simulink model "RASCAL72_cl"  (R2017b)
settings: Solver=FixedStepDiscrete  StartTime=0.0  StopTime=100  RelTol=1e-3  EnableMultiTasking=on
values from neighbouring files (symbols this model uses):
  CD0 = 0.0164    [Final_Project_START.m]
  CDa_200 = [0.53 0.53 0.53 0.53 0.53 0.53 0.53 0.53 0.53 0.53 0.53 0.53 ... (25 elements, 5x5)]    [C1o_200.mat]    (also in CDa_200.mat; CLadot_200.mat; CLde.mat; CLo_200.mat)
  CDde_200 = [0 0 0 0 0 0 0 0 0 0 0 0 ... (25 elements, 5x5)]    [C1o_200.mat]    (also in CDde_200.mat; CLadot_200.mat; CLde.mat; CLo_200.mat)
  CDq_200 = [0 0 0 0 0 0 0 0 0 0 0 0 ... (25 elements, 5x5)]    [C1o_200.mat]    (also in CDq_200.mat; CLadot_200.mat; CLde.mat; CLo_200.mat)
  CL0 = 0.21    [Final_Project_START.m]
  Cl0 = 0    [Final_Project_START.m]
  CLa_200 = [5.326215664 5.440234265 5.741037107 5.849899088 5.539928921 5.331372284 5.445390885 5.746766685 5.849899088 5.539355963 5.335955946 5.449401589 ... (25 elements, 5x5)]    [C1o_200.mat]    (also in CLa_200.mat; CLadot_200.mat; CLde.mat; CLo_200.mat)
  ClB_200 = [-0.052500123 -0.052614714 -0.052614714 -0.05294703 -0.053136106 -0.052523041 -0.052649092 -0.052666281 -0.053015785 -0.05322205 -0.052545959 -0.0525345 ... (25 elements, 5x5)]    [C1B_200.mat]    (also in C1o_200.mat; CLadot_200.mat; Cma_200.mat; Cmadot_200.mat)
  Clda_200 = [0.03678389 0.037299552 0.037299552 0.036726595 0.035580679 0.03678389 0.037299552 0.037299552 0.036726595 0.035580679 0.03678389 0.037299552 ... (25 elements, 5x5)]    [C1da_200.mat]    (also in C1o_200.mat = [0.000642 0.000651 0.000651 0.000641 0.000621 0.000642 0.000; CLadot_200.mat = [0.000642 0.000651 0.000651 0.000641 0.000621 0.000642 0.000; Cma_200.mat = [0.000642 0.000651 0.000651 0.000641 0.000621 0.000642 0.000; Cmadot_200.mat = [0.000642 0.000651 0.000651 0.000641 0.000621 0.000642 0.000)
  CLde_200 = [0.001609 0.00164 0.001639 0.001604 0.001542 0.001609 0.00164 0.001639 0.001604 0.001542 0.001609 0.00164 ... (25 elements, 5x5)]    [C1o_200.mat]    (also in CLadot_200.mat; CLde.mat; CLde_200.mat = [0.092188909 0.093965078 0.093907783 0.09190243 0.088350092 ; CLo_200.mat)
  Cldr_200 = [-5.72958e-05 0 5.72958e-05 0.000114592 0.000171887 -5.72958e-05 0 5.72958e-05 0.000114592 0.000171887 -5.72958e-05 0 ... (25 elements, 5x5)]    [C1dr_200.mat]    (also in C1o_200.mat = [-1e-06 0 1e-06 2e-06 3e-06 -1e-06 0 1e-06 2e-06 3e-06 -1e-0; CLadot_200.mat = [-1e-06 0 1e-06 2e-06 3e-06 -1e-06 0 1e-06 2e-06 3e-06 -1e-0; Cma_200.mat = [-1e-06 0 1e-06 2e-06 3e-06 -1e-06 0 1e-06 2e-06 3e-06 -1e-0; Cmadot_200.mat = [-1e-06 0 1e-06 2e-06 3e-06 -1e-06 0 1e-06 2e-06 3e-06 -1e-0)
  Clp_200 = [-0.448740545 -0.460829955 -0.490337281 -0.496124155 -0.462205053 -0.448740545 -0.460772659 -0.490279985 -0.496009563 -0.461861279 -0.448797841 -0.460829955 ... (25 elements, 5x5)]    [C1o_200.mat]    (also in C1p_200.mat; CLadot_200.mat; Cma_200.mat; Cmadot_200.mat)
  CLq_200 = [9.310564171 9.310564171 9.310564171 9.310564171 9.310564171 9.344941639 9.344941639 9.344941639 9.344941639 9.344941639 9.373589528 9.373589528 ... (25 elements, 5x5)]    [C1o_200.mat]    (also in CLadot_200.mat; CLde.mat; CLo_200.mat; CLq_200.mat)
  Clr_200 = [-0.074885584 0.016254813 0.110122488 0.213369483 0.308595068 -0.07494288 0.016260542 0.11023708 0.21354137 0.308824252 -0.075000175 0.016272001 ... (25 elements, 5x5)]    [C1o_200.mat]    (also in C1r_200.mat; CLadot_200.mat; CLde.mat; CLo_200.mat)
  Cm0 = 0    [Final_Project_START.m]
  Cma_200 = [-1.61689 -1.94061 -2.12224 -2.54508 -2.95302 -1.61918 -1.94978 -2.1314 -2.55367 -2.96506 -1.62319 -1.9578 ... (25 elements, 5x5)]    [C1o_200.mat]    (also in CLadot_200.mat; CLde.mat; CLo_200.mat; CLq_200.mat)
  Cmde_200 = [-0.002239 -0.002272 -0.00227 -0.00223 -0.002161 -0.002239 -0.002272 -0.00227 -0.00223 -0.002161 -0.002239 -0.002272 ... (25 elements, 5x5)]    [C1o_200.mat]    (also in CLadot_200.mat; CLde.mat; CLo_200.mat; CLq_200.mat)
  Cmq_200 = [-17.06841272 -17.06841272 -17.06841272 -17.06841272 -17.06841272 -17.17154512 -17.17154512 -17.17154512 -17.17154512 -17.17154512 -17.25175921 -17.25175921 ... (25 elements, 5x5)]    [C1o_200.mat]    (also in CLadot_200.mat; CLde.mat; CLo_200.mat; CLq_200.mat)
  Cn0 = 0    [Final_Project_START.m]
  CnB_200 = [0.029759428 0.029759428 0.029759428 0.029759428 0.029759428 0.028264008 0.028264008 0.028264008 0.028264008 0.028264008 0.027209766 0.027209766 ... (25 elements, 5x5)]    [C1o_200.mat]    (also in CLadot_200.mat; CLde.mat; CLo_200.mat; CLq_200.mat)
  Cnda_200 = [-4.5e-05 -2.9e-05 -1.1e-05 6e-06 2.2e-05 -4.5e-05 -2.9e-05 -1.1e-05 6e-06 2.2e-05 -4.5e-05 -2.9e-05 ... (25 elements, 5x5)]    [C1o_200.mat]    (also in CLadot_200.mat; CLde.mat; CLo_200.mat; CLq_200.mat)
  Cndr_200 = [0.000151 0.000159 0.000163 0.000164 0.00016 0.000151 0.000159 0.000163 0.000164 0.00016 0.000151 0.000159 ... (25 elements, 5x5)]    [C1o_200.mat]    (also in CLadot_200.mat; CLde.mat; CLo_200.mat; CLq_200.mat)
  Cnp_200 = [0.038193 0.000534 -0.03759 -0.07993 -0.12032 0.039712 0.000373 -0.03967 -0.08394 -0.12594 0.040583 0.00028 ... (25 elements, 5x5)]    [C1o_200.mat]    (also in CLadot_200.mat; CLde.mat; CLo_200.mat; CLq_200.mat)
  Cnr_200 = [-0.040473739 -0.043229666 -0.042771299 -0.038405361 -0.030859507 -0.040015372 -0.042908809 -0.042244178 -0.037247986 -0.028751022 -0.039728894 -0.042702544 ... (25 elements, 5x5)]    [C1o_200.mat]    (also in CLadot_200.mat; CLde.mat; CLo_200.mat; CLq_200.mat)
  CY0 = 0    [Final_Project_START.m]
  CYB_200 = [-0.504374747 -0.504374747 -0.504374747 -0.504374747 -0.504374747 -0.504374747 -0.504374747 -0.504374747 -0.504374747 -0.504374747 -0.504432043 -0.50432043 ... (25 elements, 5x5)]    [C1o_200.mat]    (also in CLadot_200.mat; CLde.mat; CLo_200.mat; CLq_200.mat)
  CYda_200 = [4e-06 2.7e-05 5e-05 7.1e-05 9.1e-05 4e-06 2.7e-05 5e-05 7.1e-05 9.1e-05 4e-06 2.7e-05 ... (25 elements, 5x5)]    [C1o_200.mat]    (also in CLadot_200.mat; CLde.mat; CLo_200.mat; CLq_200.mat)
  CYdr_200 = [-0.000731 -0.000766 -0.000782 -0.00078 -0.000759 -0.000731 -0.000766 -0.000782 -0.00078 -0.000759 -0.000731 -0.000766 ... (25 elements, 5x5)]    [C1o_200.mat]    (also in CLadot_200.mat; CLde.mat; CLo_200.mat; CLq_200.mat)
  CYp_200 = [-0.030521462 -0.058498991 -0.087204176 -0.119576292 -0.14919821 -0.029782346 -0.058613582 -0.088178205 -0.121581644 -0.152005703 -0.029358357 -0.058670878 ... (25 elements, 5x5)]    [C1o_200.mat]    (also in CLadot_200.mat; CLde.mat; CLo_200.mat; CLq_200.mat)
  CYr_200 = [0.026877 0.03248 0.035656 0.0363 0.03441 0.026877 0.03248 0.035656 0.0363 0.03441 0.026877 0.03248 ... (25 elements, 5x5)]    [C1o_200.mat]    (also in CLadot_200.mat; CLde.mat; CLo_200.mat; CLq_200.mat)
undefined symbols (not defined in the file or in its folder): airlib, B747, DiscIntNeverNeededParam, DT
(part 1 of 2)
settings Model: Creator=SHETTYA1  LastModifiedBy=antar
settings DataIOCC: SaveFormat=Array  SignalLoggingSaveFormat=ModelDataLogs  SaveOutput=off  SaveTime=off
settings OptimizationCC: BlockReduction=off  BooleanDataType=off
settings DebuggingCC: SaveWithParameterizedLinksMsg=none  UnderspecifiedInitializationDetection=Classic  MergeDetectMultiDrivingBlocksExec=none  SignalResolutionControl=TryResolveAllWithWarning  MultiTaskDSMMsg=warning  MultiTaskCondExecSysMsg=none
settings HardwareCC: TargetUnknown=on
settings ModelReferenceCC: PropagateSignalLabelsOutOfModel=off
settings CodeAppCC: StateflowObjectComments=on
settings GRTTargetCC: TargetLangStandard=C89/C90 (ANSI)  CombineOutputUpdateFcns=off  GRTInterface=on

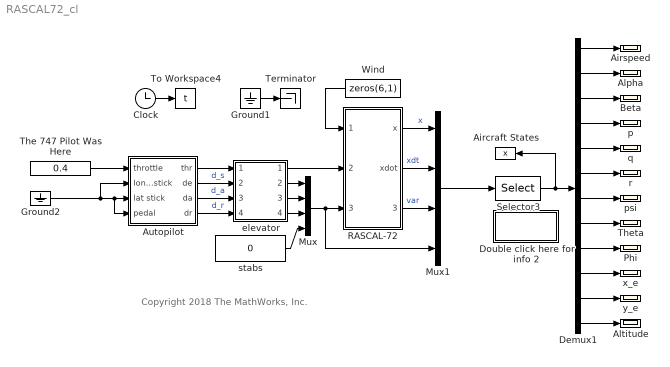
== system RASCAL72_cl ==
  note: Copyright 2018 The MathWorks, Inc.
  Aircraft States : ToWorkspace  VariableName=x  SampleTime=0.05
  Airspeed : Scope
  Alpha : Scope
  Altitude : Scope
  Autopilot : Subsystem
  Beta : Scope
  Clock : Clock
  Demux1 : Demux  Outputs=12
  Double click here for info 2 : Subsystem
      mask Display: disp('Output\nSignals')
  Ground1 : Ground
  Ground2 : Ground
  Mux : Mux
  Mux1 : Mux  Inputs=[12 12 12 4]
  Phi : Scope
  RASCAL-72 : Subsystem  AncestorBlock=airlib/DT-B747  mask(Discrete Time General Nonlinear Aircraft Model){GM1=[0.244   1.84   0.327418   1.7398  1.3865   1.7122   0   0  0   2.9  0.05], CD_wind=[0.076   0.53  0  0  0], CL_wind=[0.2  5.849899088  9.310  0.001604  0], Cm_body=[0.3567  -2.54508  -17.0684   -7.288023154    0], CY_body=[0   -0.504374747  -0.119633588   0.0363     0.000071  -0.00078  ], Cl_body=[0  -0.05294703   -0.496124155    0.213369  0.000641  0.000002], Cn_body=[0 0.029747969 -0.07993 -0.038399631 0.000006 0.000164], x0=[10 0.0264  0   0 0 0   0  0.08  0   0 0 100]}
      mask prompts: GM1 "Geometry, Mass, T : [cbar   b    S    Ix   Iy   Iz   Jxy  Jxz  Jyz  m  T]"; CD_wind "Aerodynamic D-Force Derivatives : [CD0 CDa CDq CDde CDih]"; CL_wind "Aerodynamic L-Force Derivatives : [CL0 CLa CLq CLde CLih]"; Cm_body "Aerodynamic Y-Moment Derivatives : [Cm0 Cma Cmq Cmde Cmih]"; CY_body "Aerodynamic Y-Force Derivatives : [CY0 CYb CYp CYr CYda CYdr]"; Cl_body "Aerodynamic X-moment Derivatives : [Cl0 Clb Clp Clr Clda Cldr]"; Cn_body "Aerodynamic Z-moment Derivatives : [Cn0 Cnb Cnp Cnr Cnda Cndr]"; x0 "Initial Condition x0 [v alpha beta p q r psi theta phi xe ye H]"
      mask help:
      | The first input contains the wind velocity and acceleration.The second input contains external forces and moments in body axis. The third input contains the deflections of elevators, ailerons, rudder, and flaps. For explanations about outputs and parameters open the help and/or look under the mask.
      | The International measurement system (MKS) is adopted.
      mask init:
      | AM=zeros(6,19);
      | AM(1,[1 2 9 11 12])=reshape(CD_wind,1,5);
      | AM(3,[1 2 9 11 12])=reshape(CL_wind,1,5);
      | AM(5,[1 2 9 11 12])=reshape(Cm_body,1,5);
      | AM(2,[1 5 8 10 13 14])=reshape(CY_body,1,6);
      | AM(4,[1 5 8 10 13 14])=reshape(Cl_body,1,6);
      | AM(6,[1 5 8 10 13 14])=reshape(Cn_body,1,6);
      | 
      | Ix=GM1(4);Iy=GM1(5);Iz=GM1(6);
      | Jxy=GM1(7);Jxz=GM1(8);Jyz=GM1(9);
      | 
      | detI = Ix*Iy*Iz - 2*Jxy*Jxz*Jyz - Ix*Jyz^2 - Iy*Jxz^2 - Iz*Jxy^2;
      | I1   = Iy*Iz - Jyz^2;I2   = Jxy*Iz + Jyz*Jxz;
      | I3   = Jxy*Jyz + Iy*Jxz;I4   = Ix*Iz - Jxz^2;
      | I5   = Ix*Jyz + Jxy*Jxz;I6   = Ix*Iy - Jxy^2;
      | 
      | Pl  = I1/detI; Pm = I2/detI; Pn = I3/detI;
      | Ppp = -(Jxz*I2 - Jxy*I3)/detI;Ppq = (Jxz*I1 - Jyz*I2 - (Iy-Ix)*I3)/detI;
      | Ppr = -(Jxy*I1 + (Ix-Iz)*I2 - Jyz*I3)/detI;Pqq = (Jyz*I1 - Jxy*I3)/detI;
      | Pqr = -((Iz-Iy)*I1 - Jxy*I2 + Jxz*I3)/detI;Prr = -(Jyz*I1 - Jxz*I2)/detI;
      | 
      | Ql  = I2/detI; Qm = I4/detI; Qn = I5/detI;
      | Qpp = -(Jxz*I4 - Jxy*I5)/detI;Qpq = (Jxz*I2 - Jyz*I4 - (Iy-Ix)*I5)/detI;
      | Qpr = -(Jxy*I2 + (Ix-Iz)*I4 - Jyz*I5)/detI;Qqq = (Jyz*I2 - Jxy*I5)/detI;
      | Qqr = -((Iz-Iy)*I2 - Jxy*I4 + Jxz*I5)/detI;Qrr = -(Jyz*I2 - Jxz*I4)/detI;
      | 
      | Rl  = I3/detI; Rm = I5/detI; Rn = I6/detI;
      | Rpp = -(Jxz*I5 - Jxy*I6)/detI;
      | Rpq = (Jxz*I3 - Jyz*I5 - (Iy-Ix)*I6)/detI;
      | Rpr = -(Jxy*I3 + (Ix-Iz)*I5 - Jyz*I6)/detI;
      | Rqq = (Jyz*I3 - Jxy*I6)/detI;
      | Rqr = -((Iz-Iy)*I3 - Jxy*I5 + Jxz*I6)/detI;
      | Rrr = -(Jyz*I3 - Jxz*I5)/detI;
      | 
      | GM2 = [  Pl   Pm   Pn   Ppp  Ppq  Ppr  Pqq  Pqr  Prr ;
      |                Ql  Qm   Qn   Qpp  Qpq  Qpr  Qqq  Qqr  Qrr ;
      |                Rl  Rm   Rn   Rpp  Rpq  Rpr  Rqq  Rqr  Rrr ];
      | 
      | xfix=1;
      | T=GM1(11);
      mask Help:
      | <p>
      | This block is a general nonlinear 6DOF aircraft model, with a very accurate built-in atmosphere model and constant aerodynamic derivatives.
      | The architecture of the block is largely based on the Aircraft block provided by the <A
      | HREF="http://www.mathworks.com/matlabcentral/fileexchange/loadFile.do?objectId=252&objectType=file">FDC toolbox</A> (Marc Rauw, 1993-2000).
      | </p>
      | <p>
      | The geometric and inertal data of the aircraft are entered as parameters in the first row of the mask, sampling time is the last parameter. The other six rows contains the non-dimensional aerodynamic derivatives. The last row is the initial state.
      | </p>
      | <p>
      | The first input contains the wind velocity and acceleration.
      | The second input contains external forces and moments in the aircraft body axis.
      | The third input contains the deflections of elevators, ailerons, rudder,
      | and flaps or stabilators. For a list of outputs look under the mask.
      | </p>
      | <p>
      | The control surface sign conventions are the same adopted in books such as Stevens-Lewis and Etkin, and in many flight simulators,
      | including the FDC toolbox. <br>
      | Specifically, positive elevator deflection causes negative pitching moment (Cmde &#60 0), positive rudder deflection causes negative yawing
      | moment (Cndr &#60 0), and positive aileron deflection causes negative rolling moment (Clda &#60 0). Another way to say the same thing is
      | that, the positive elevators deflection is Trailing Edge Down (TED), the positive rudder(s) deflection is Trailing Edge Left (TEL), and,
      | taking as TED the positive ailerons deflection, da=K*(da_right-da_left), with K usually equal to 1 (FDC) or 1/2.
      | </p>
      | <p>
      | Since this block is largely based on the FDC toolbox, i redirect you to the FDC Toolbox manual, for a good explanation of the underlying
      | components. Besides the mask and the fact that the aerodynamic derivatives are expressed in the stability axis, the only relevant difference
      | with the FDC toolbox is that in the computation of the aerodynamic forces, q is normalized as q*cbar/2V instead of q*cbar/V. The majority
      | of aeronautics books that i've seen use q*cbar/2V.
      | </p>
      | <p>
      | Please note that the International Measurement System is adopted. So, lengths are in meters, masses in Kg, and inertia moments in Kg*m^2.
      | Moreover, forces are in N, moments in N*m, accelerations in g, and angles in radians. For those that use the english system, here are some useful
      | conversion factors: <br>
      | 1 ft   = 0.3048 m, 1 lb   = 0.4536 Kg, 1 slug = 14.593903 Kg ,  1 slug*ft^2 = 1.355818 Kg*m^2
      | <br>
      | </p>
      | <p>
      | Finally, there is an <A HREF="http://www.aae.uiuc.edu/m-selig/apasim/Aircraft-uiuc.html">excellent source</A> of aircraft aerodynamic data
      | which is mantained by Michael S. Selig, Rob Deters, and Glen Dimock at the university of Urbana-Champaign. To use any of the given models
      | you just need to type the supplied aircraft data in the block mask.
      | </p>
      | <p>
      | <p>
      | December 2002, Giampiero Campa
      | </p>
      | </p>
      mask Display: disp('Discrete\nTime\nGeneral\nAircraft\nModel')
  Selector3 : Selector  InputPortWidth=40  IndexOptions=Index vector (dialog)  Indices=1:12  OutputSizes=1
  Terminator : Terminator
  The 747 Pilot Was Here : Constant  Value=0.4
  Theta : Scope
  To Workspace4 : ToWorkspace  VariableName=t  SampleTime=0.05
  Wind : Constant  Value=zeros(6,1)
  elevator : Subsystem
      mask Display: disp('Cable &\nactuator\ndynamics')
  p : Scope
  psi : Scope
  q : Scope
  r : Scope
  stabs : Constant  Value=0
  x_e : Scope
  y_e : Scope
  wires:
  elevator/3(deltaa) -> Mux/2
  elevator/4(deltar) -> Mux/3
  elevator/2(deltae) -> Mux/1
  Autopilot/2(de) -> elevator/2(D_elv)  "d_s"
  Autopilot/3(da) -> elevator/3(D_ail)  "d_a"
  Autopilot/4(dr) -> elevator/4(D_rud)  "d_r"
  Mux/1 -> Mux1/4, RASCAL-72/3(deflect)
  elevator/1(throttle) -> RASCAL-72/2(ext fm)
  Mux1/1 -> Selector3/1
  Selector3/1 -> Demux1/1, Aircraft States/1
  Demux1/1 -> Airspeed/1
  Demux1/2 -> Alpha/1
  Demux1/3 -> Beta/1
  Demux1/4 -> p/1
  Demux1/5 -> q/1
  Demux1/6 -> r/1
  Demux1/7 -> psi/1
  Demux1/8 -> Theta/1
  Demux1/9 -> Phi/1
  Demux1/10 -> x_e/1
  Demux1/11 -> y_e/1
  Demux1/12 -> Altitude/1
  Autopilot/1(thr) -> elevator/1(D_thr)
  Clock/1 -> To Workspace4/1
  stabs/1 -> Mux/4
  Wind/1 -> RASCAL-72/1(" uwind")
  RASCAL-72/1(x) -> Mux1/1  "x"
  RASCAL-72/2(xdot) -> Mux1/2  "xdt"
  RASCAL-72/3(others) -> Mux1/3  "var"
  The 747 Pilot Was Here/1 -> Autopilot/1(throttle)
  Ground2/1 -> Autopilot/3(lat stick), Autopilot/4(pedal), Autopilot/2(long stick)
  Ground1/1 -> Terminator/1

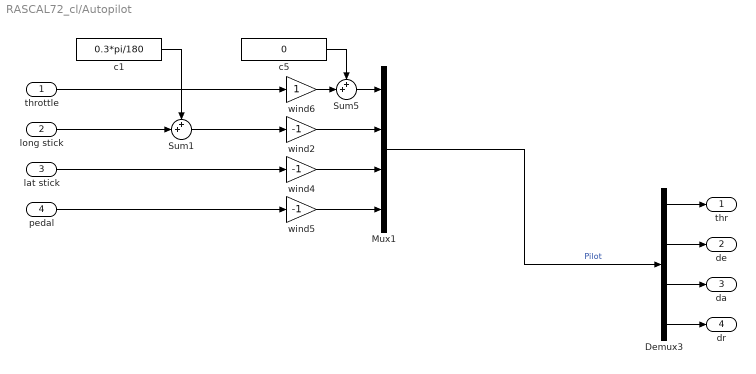
== system RASCAL72_cl/Autopilot ==
  throttle : Inport
  long stick : Inport  Port=2
  lat stick : Inport  Port=3
  pedal : Inport  Port=4
  Demux3 : Demux
  Mux1 : Mux
  Sum1 : Sum  Inputs=++|  SaturateOnIntegerOverflow=on  InputSameDT=on  OutDataTypeStr=Inherit: Same as first input
  Sum5 : Sum  Inputs=++|  SaturateOnIntegerOverflow=on  InputSameDT=on  OutDataTypeStr=Inherit: Same as first input
  c1 : Constant  Value=0.3*pi/180
  c5 : Constant  Value=0
  wind2 : Gain  Gain=-1  SaturateOnIntegerOverflow=on  OutDataTypeStr=Inherit: Same as input  ParamDataTypeStr=Inherit: Same as input
  wind4 : Gain  Gain=-1  SaturateOnIntegerOverflow=on  OutDataTypeStr=Inherit: Same as input  ParamDataTypeStr=Inherit: Same as input
  wind5 : Gain  Gain=-1  SaturateOnIntegerOverflow=on  OutDataTypeStr=Inherit: Same as input  ParamDataTypeStr=Inherit: Same as input
  wind6 : Gain  SaturateOnIntegerOverflow=on  OutDataTypeStr=Inherit: Same as input  ParamDataTypeStr=Inherit: Same as input
  thr : Outport
  de : Outport  Port=2
  da : Outport  Port=3
  dr : Outport  Port=4
  wires:
  lat stick/1 -> wind4/1
  pedal/1 -> wind5/1
  Mux1/1 -> Demux3/1  "Pilot"
  Demux3/1 -> thr/1
  Demux3/2 -> de/1
  Demux3/3 -> da/1
  Demux3/4 -> dr/1
  wind2/1 -> Mux1/2
  wind4/1 -> Mux1/3
  wind5/1 -> Mux1/4
  Sum5/1 -> Mux1/1
  throttle/1 -> wind6/1
  c5/1 -> Sum5/1
  wind6/1 -> Sum5/2
  long stick/1 -> Sum1/2
  Sum1/1 -> wind2/1
  c1/1 -> Sum1/1

== system RASCAL72_cl/Double click here for info 2 ==
  note: 01 v (m/s)
      | 02 alpha (rad)
      | 03 beta (rad)
      | 04 p (rad/s)
      | 05 q (rad/s)
      | 06 r  (rad/s)
      | 07 psi (rad)
      | 08 theta (rad)
      | 09 phi (rad)
      | 10 xe (m)
      | 11 ye (m)
      | 12 ze (m)
      | 13 v dot (m/s2)
      | 14 alpha dot (rad/s)
      | 15 beta dot (rad/s)
      | 16 p dot (rad/s2)
      | 17 q dot (rad/s2)
      | 18 r dot (rad/s2)
      | 19 fi dot (rad/s)
      | 20 theta dot (rad/s)
      | 21 psi dot (rad/s)
      | 22 xe dot (m/s)
      | 23 ye dot (m/s)
      | 24 ze dot (m/s)
      | 25 u dot (m/s2)
      | 26 v dot (m/s2)
      | 27 w dot (m/s2)
      | 28 pb/2v (rad)
      | 29 qc/v (rad)
      | 30 rb/v (rad)
      | 31 Ax (g)
      | 32 Ay (g)
      | 33 Az (g)
      | 34 ax (g)
      | 35 ay (g)
      | 36 az (g)
      | 37 delta elevators (rad)
      | 38 delta ailerons (rad)
      | 39 delta rudder (rad)
      | 40 delta stabs (rad)

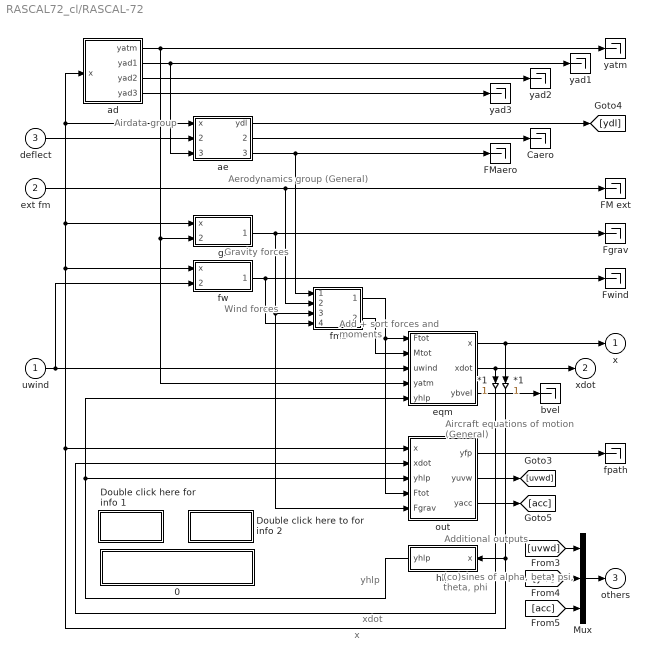
== system RASCAL72_cl/RASCAL-72 ==
  note: Airdata group
  note: Add + sort
      | forces and
      | moments
  note: (co)sines of
      | alpha, beta,
      | psi, theta, phi
  note: Aerodynamics
      | group (General)
  note: Gravity forces
  note: Wind forces
  note: Aircraft equations
      | of motion (General)
  note: Additional outputs
  note: yhlp
  note: x
  note: xdot
  " uwind" : Inport
  ext fm : Inport  Port=2
  deflect : Inport  Port=3
  " *1" : Gain  SaturateOnIntegerOverflow=on  OutDataTypeStr=Inherit: Same as input  ParamDataTypeStr=Inherit: Same as input
  *1 : Gain  SaturateOnIntegerOverflow=on  OutDataTypeStr=Inherit: Same as input  ParamDataTypeStr=Inherit: Same as input
  0 : Subsystem
      mask Display: disp('AIRCRAFT, main level\nM.O. Rauw')
  Caero : Terminator
  Double click here for info 1 : Subsystem
      mask Display: disp('Input\nSignals')
  Double click here to for info 2 : Subsystem
      mask Display: disp('Output\nSignals')
  FM ext : Terminator
  FMaero : Terminator
  Fgrav : Terminator
  Fwind : Terminator
  Mux : Mux  Inputs=[3 3 6]
  ad : Subsystem
  ae : Subsystem
  bvel : Terminator
  eqm : Subsystem
  fms : Subsystem  mask(FMsort){}
      mask help: Forces and Moments sorting block
      mask Display: disp('FMsort')
  fpath : Terminator
  fw : Subsystem  mask(fwind){m=GM1(10)}
      mask prompts: m "Mass of the aircraft [kg]:"
      mask help: Forces due to non-steady atmosphere.
      mask Display: disp('Fwind')
  gr : Subsystem  mask(Gravity){m=GM1(10)}
      mask prompts: m "Mass of the aircraft [kg]:"
      mask help: Gravity forces.
      mask Display: disp('Gravity')
  hlp : Subsystem  mask(Hlpfcn){}
      mask help: Help sines and cosines
      mask Display: disp('hlpfcn')
  out : Subsystem
  yad1 : Terminator
  yad2 : Terminator
  yad3 : Terminator
  yatm : Terminator
  x : Outport
  xdot : Outport  Port=2
  others : Outport  Port=3
  wires:
  Mux/1 -> others/1
  [acc] -> Mux/3
  [ydl] -> Mux/2
  [uvwd] -> Mux/1
  out/2(yuvw) -> [uvwd]
  fms/2(Mtot) -> eqm/2(Mtot)
  eqm/1(x) -> " *1"/1, x/1
  eqm/2(xdot) -> *1/1, xdot/1
  " *1"/1 -> ad/1(x), ae/1(x), gr/1(x), fw/1(x), out/1(x), hlp/1(x)
  gr/1(Fgrav) -> Fgrav/1, out/5(Fgrav), fms/3(Fgrav)
  *1/1 -> out/2(xdot)
  " uwind"/1 -> fw/2(uwind), eqm/3(uwind)
  hlp/1(yhlp) -> out/3(yhlp), eqm/5(yhlp)
  ae/3(FMaero) -> fms/1(FMaero), FMaero/1
  fw/1(Fwind) -> fms/4(Fwind), Fwind/1
  out/3(yacc) -> [acc]
  ad/1(yatm) -> yatm/1, gr/2(yatm), eqm/4(yatm)
  ad/3(yad2) -> yad2/1
  ad/2(yad1) -> yad1/1, ae/3(yad1)
  out/1(yfp) -> fpath/1
  eqm/3(ybvel) -> bvel/1
  ae/2(Caero) -> Caero/1
  ae/1(ydl) -> [ydl]
  ad/4(yad3) -> yad3/1
  deflect/1 -> ae/2(uaero)
  ext fm/1 -> FM ext/1, fms/2(FMprop)
  fms/1(Ftot) -> eqm/1(Ftot), out/4(Ftot)

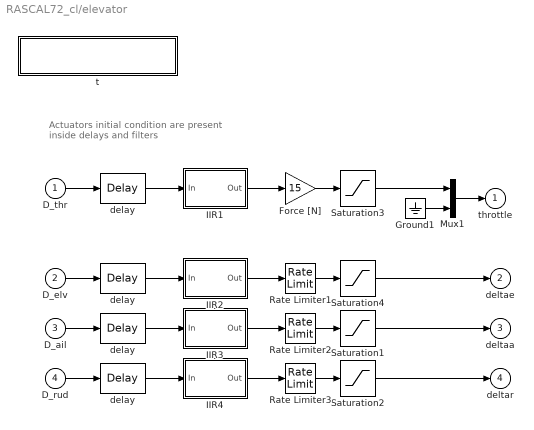
== system RASCAL72_cl/elevator ==
  note: Actuators initial condition are present
      | inside delays and filters
  D_thr : Inport
  D_elv : Inport  Port=2
  D_ail : Inport  Port=3
  D_rud : Inport  Port=4
  " delay" : TransportDelay  DelayTime=0.03  InitialOutput=-1.71374e-004
  " delay " : TransportDelay  DelayTime=0.03  InitialOutput=0.490154
  Force [N] : Gain  Gain=15  SaturateOnIntegerOverflow=on  OutDataTypeStr=Inherit: Same as input  ParamDataTypeStr=Inherit: Same as input
  Ground1 : Ground
  IIR1 : Subsystem  mask(Discrete Time First Order IIR){ni=1, a=4, x0=0.490154, T=0.05}
      mask prompts: ni "Number of Channels"; a "Cutoff Frequency (a)"; x0 "Initial Condition"; T "Sample Time"
      mask help:
      | Each channel has the transfer function
      |   (1-exp(-aT))/(1-exp(-aT)(z^-1)) which is a good
      |   (pz-matched) approximation of a/(s+a) if 10*a*T<pi
      mask init:
      | A=[];B=[];C=[];D=[];
      | for i=1:ni,
      | A=[A,zeros(size(A,1),1);zeros(1,size(A,2)),exp(-a*T)];
      | B=[B,zeros(size(B,1),1);zeros(1,size(B,2)),1-exp(-a*T)];
      | C=[C,zeros(size(C,1),1);zeros(1,size(C,2)),exp(-a*T)];
      | D=[D,zeros(size(D,1),1);zeros(1,size(D,2)),1-exp(-a*T)];
      | end
      mask Help:
      | <p>
      |   Each channel has the transfer function
      |   (1-exp(-aT))/(1-exp(-aT)(z^-1)) which is a good
      |   (pz-matched) approximation of a/(s+a) if 10*a*T<pi
      | </p>
      mask Display: dpoly(a,[1 a],'s')
  IIR2 : Subsystem  mask(Discrete Time First Order IIR){ni=1, a=15, x0=-1.71374e-004, T=0.05}
      mask prompts: ni "Number of Channels"; a "Cutoff Frequency (a)"; x0 "Initial Condition"; T "Sample Time"
      mask help:
      | Each channel has the transfer function
      |   (1-exp(-aT))/(1-exp(-aT)(z^-1)) which is a good
      |   (pz-matched) approximation of a/(s+a) if 10*a*T<pi
      mask init: same as RASCAL72_cl/elevator/IIR1
      mask Help:
      | <p>
      |   Each channel has the transfer function
      |   (1-exp(-aT))/(1-exp(-aT)(z^-1)) which is a good
      |   (pz-matched) approximation of a/(s+a) if 10*a*T<pi
      | </p>
      mask Display: dpoly(a,[1 a],'s')
  IIR3 : Subsystem  mask(Discrete Time First Order IIR){ni=1, a=40, x0=0, T=0.05}
      mask prompts: ni "Number of Channels"; a "Cutoff Frequency (a)"; x0 "Initial Condition"; T "Sample Time"
      mask help:
      | Each channel has the transfer function
      |   (1-exp(-aT))/(1-exp(-aT)(z^-1)) which is a good
      |   (pz-matched) approximation of a/(s+a) if 10*a*T<pi
      mask init: same as RASCAL72_cl/elevator/IIR1
      mask Help:
      | <p>
      |   Each channel has the transfer function
      |   (1-exp(-aT))/(1-exp(-aT)(z^-1)) which is a good
      |   (pz-matched) approximation of a/(s+a) if 10*a*T<pi
      | </p>
      mask Display: dpoly(a,[1 a],'s')
  IIR4 : Subsystem  mask(Discrete Time First Order IIR){ni=1, a=15, x0=0, T=0.05}
      mask prompts: ni "Number of Channels"; a "Cutoff Frequency (a)"; x0 "Initial Condition"; T "Sample Time"
      mask help:
      | Each channel has the transfer function
      |   (1-exp(-aT))/(1-exp(-aT)(z^-1)) which is a good
      |   (pz-matched) approximation of a/(s+a) if 10*a*T<pi
      mask init: same as RASCAL72_cl/elevator/IIR1
      mask Help:
      | <p>
      |   Each channel has the transfer function
      |   (1-exp(-aT))/(1-exp(-aT)(z^-1)) which is a good
      |   (pz-matched) approximation of a/(s+a) if 10*a*T<pi
      | </p>
      mask Display: dpoly(a,[1 a],'s')
  Mux1 : Mux  Inputs=[1 5]
  Rate Limiter1 : RateLimiter  RisingSlewLimit=100*pi/180  FallingSlewLimit=-100*pi/180
  Rate Limiter2 : RateLimiter  RisingSlewLimit=100*pi/180  FallingSlewLimit=-100*pi/180
  Rate Limiter3 : RateLimiter  RisingSlewLimit=100*pi/180  FallingSlewLimit=-100*pi/180
  Saturation1 : Saturate  UpperLimit=20*pi/180  LowerLimit=-20*pi/180
  Saturation2 : Saturate  UpperLimit=20*pi/180  LowerLimit=-20*pi/180
  Saturation3 : Saturate  UpperLimit=245440  LowerLimit=0
  Saturation4 : Saturate  UpperLimit=20*pi/180  LowerLimit=-20*pi/180
  delay : TransportDelay  DelayTime=0.03
  "delay " : TransportDelay  DelayTime=0.03
  t : Subsystem
      settings: OpenFcn=fdchelp actuatr
      mask Display: disp('Actuator & cable dynamics\nMarc Rauw, October 1997')
  throttle : Outport
  deltae : Outport  Port=2
  deltaa : Outport  Port=3
  deltar : Outport  Port=4
  wires:
  D_ail/1 -> delay/1
  D_elv/1 -> " delay"/1
  D_rud/1 -> "delay "/1
  IIR2/1(Out) -> Rate Limiter1/1
  Saturation4/1 -> deltae/1
  IIR3/1(Out) -> Rate Limiter2/1
  Saturation1/1 -> deltaa/1
  IIR4/1(Out) -> Rate Limiter3/1
  Saturation2/1 -> deltar/1
  Rate Limiter1/1 -> Saturation4/1
  Rate Limiter2/1 -> Saturation1/1
  Rate Limiter3/1 -> Saturation2/1
  Mux1/1 -> throttle/1
  Saturation3/1 -> Mux1/1
  Ground1/1 -> Mux1/2
  D_thr/1 -> " delay "/1
  IIR1/1(Out) -> Force [N]/1
  Force [N]/1 -> Saturation3/1
  " delay "/1 -> IIR1/1(In)
  " delay"/1 -> IIR2/1(In)
  delay/1 -> IIR3/1(In)
  "delay "/1 -> IIR4/1(In)

== system RASCAL72_cl/RASCAL-72/0 ==

== system RASCAL72_cl/RASCAL-72/Double click here for info 1 ==
  note: 01 Uwind (m/s)
      | 02 Vwind (m/s)
      | 03 Wwind (m/s)
      | 04 Uwind_dot (m/s2)
      | 05 Vwind_dot (m/s2)
      | 06 Wwind_dot (m/s2)
      |
      | 07 Fx (N)
      | 08 Fy (N)
      | 09 Fz (N)
      | 10 Mx (N)
      | 11 My (N)
      | 12 Mz (N)
      |
      | 13 delta elevators (rad)
      | 14 delta ailerons (rad)
      | 15 delta rudder (rad)
      | 16 delta stabs/flaps (rad)

== system RASCAL72_cl/RASCAL-72/Double click here to for info 2 ==
  note: 01 v (m/s)
      | 02 alpha (rad)
      | 03 beta (rad)
      | 04 p (rad/s)
      | 05 q (rad/s)
      | 06 r  (rad/s)
      | 07 psi (rad)
      | 08 theta (rad)
      | 09 phi (rad)
      | 10 xe (m)
      | 11 ye (m)
      | 12 ze (m)
      |
      | 13 v dot (m/s2)
      | 14 alpha dot (rad/s)
      | 15 beta dot (rad/s)
      | 16 p dot (rad/s2)
      | 17 q dot (rad/s2)
      | 18 r dot (rad/s2)
      | 19 fi dot (rad/s)
      | 20 theta dot (rad/s)
      | 21 psi dot (rad/s)
      | 22 xe dot (m/s)
      | 23 ye dot (m/s)
      | 24 ze dot (m/s)
      |
      | 25 u dot (m/s2)
      | 26 v dot (m/s2)
      | 27 w dot (m/s2)
      | 28 pb/2v (rad)
      | 29 qc/v (rad)
      | 30 rb/v (rad)
      | 31 Ax (g)
      | 32 Ay (g)
      | 33 Az (g)
      | 34 ax (g)
      | 35 ay (g)
      | 36 az (g)

== system RASCAL72_cl/RASCAL-72/ad ==
  x : Inport
  0 : Subsystem
      mask Display: disp('AIRDATA GROUP (level 3)\nM.O. Rauw')
  ad1 : Subsystem  mask(Airdata1){}
      mask help: Basic airdata variables
      mask Display: disp('Airdata1')
  ad2 : Subsystem  mask(Airdata2){}
      mask help: More airdata variables
      mask Display: disp('Airdata2')
  ad3 : Subsystem  mask(Airdata3){cbar=GM1(1)}
      mask prompts: cbar "Mean aerodynamic chord [m]:"
      mask help: More airdata variables
      mask Display: disp('Airdata3')
  atm : Subsystem  mask(Atmosph){}
      mask help: Atmosphere variables
      mask Display: disp('Atmosph')
  yatm : Outport
  yad1 : Outport  Port=2
  yad2 : Outport  Port=3
  yad3 : Outport  Port=4
  wires:
  ad1/1(yad1) -> ad3/3(yad1), ad2/2(yad1), yad1/1
  atm/1(yatm) -> ad3/2(yatm), ad2/1(yatm), ad1/2(yatm), yatm/1
  x/1 -> ad3/1(x), ad1/1(x), atm/1(x)
  ad3/1(yad3) -> yad3/1
  ad2/1(yad2) -> yad2/1

== system RASCAL72_cl/RASCAL-72/ae ==
  x : Inport
  uaero : Inport  Port=2
  yad1 : Inport  Port=3
  0 : Subsystem
      mask Display: disp('AERODYNAMICS GROUP (level 3)\nM.O. Rauw')
  aero : Subsystem  mask(Aeromod){}
      mask help: Aerodynamic model of the DHC-2 'Beaver'.
      mask Display: disp('Aeromod\n(General)')
  dl : Subsystem  mask(Dimless){cbar=GM1(1), b=GM1(2)}
      mask prompts: cbar "Mean aerodynamic chord [m]:"; b "Wing span [m]:"
      mask help: Dimensionless rotational velocities.
      mask Display: disp('Dimless')
  fmdims : Subsystem  mask(FMdims){cbar=GM1(1), b=GM1(2), S=GM1(3)}
      mask prompts: cbar "Mean aerodynamic chord [m]:"; b "Wing span [m]:"; S "Wing surface [m^2]:"
      mask help:
      | Calculate forces and moments from
      | dimensionless derivatives.
      mask Display: disp('FMdims')
  ydl : Outport
  Caero : Outport  Port=2
  FMaero : Outport  Port=3
  wires:
  fmdims/1(Forces and moments) -> FMaero/1
  uaero/1 -> aero/2(uaero)
  x/1 -> aero/1(x), dl/1(x)
  dl/1(ydl) -> aero/3(ydl), ydl/1
  aero/1(Caero) -> Caero/1, fmdims/2(Force / moment derivatives)
  yad1/1 -> aero/4(yad1), fmdims/1(yad1)

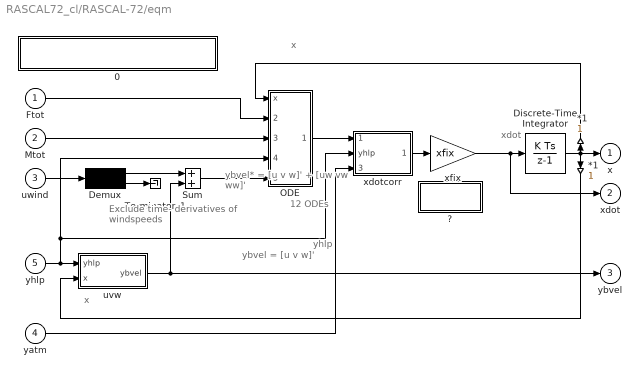
== system RASCAL72_cl/RASCAL-72/eqm ==
  note: 12 ODEs
  note: ybvel = [u v w]'
  note: yhlp
  note: x
  note: x
  note: xdot
  note: ybvel* =
      | [u v w]' +
      | [uw vw ww]'
  note: Exclude time-
      | derivatives
      | of windspeeds
  Ftot : Inport
  Mtot : Inport  Port=2
  uwind : Inport  Port=3
  yatm : Inport  Port=4
  yhlp : Inport  Port=5
  " *1" : Gain  SaturateOnIntegerOverflow=on  OutDataTypeStr=Inherit: Same as input  ParamDataTypeStr=Inherit: Same as input
  *1 : Gain  SaturateOnIntegerOverflow=on  OutDataTypeStr=Inherit: Same as input  ParamDataTypeStr=Inherit: Same as input
  0 : Subsystem
      mask Display: disp('EQUATIONS OF MOTION (level 3)\nM.O. Rauw')
  "?" : Subsystem
      mask Display: disp('More info\nfor xfix')
  Demux : Demux  Outputs=[3 3]
  Discrete-Time Integrator : DiscreteIntegrator  InitialCondition=x0  SampleTime=T  ICPrevOutput=DiscIntNeverNeededParam  ICPrevScaledInput=DiscIntNeverNeededParam
  ODE : Subsystem
  Sum : Sum  SaturateOnIntegerOverflow=on  InputSameDT=on  OutDataTypeStr=Inherit: Same as first input
  Terminator_1 : Terminator
  uvw : Subsystem  mask(uvw){}
      mask help:
      | Calculation of body-axes velocities
      | u, v, and w
      mask Display: disp('Body-axes\nvelocities')
  xdotcorr : Subsystem  mask(xdotcorr){b=GM1(2), S=GM1(3), m=GM1(10), CYbdot=AM(2,19)}
      mask prompts: b "Wing span [m]:"; S "Wing surface [m^2]:"; m "Mass of the aircraft [kg]:"; CYbdot "Stability-derivative CYbdot:"
      mask help:
      | Correction block to write state
      | equations for DHC-2 Beaver aircraft
      | explicitly.
      mask Display: disp('xdotcorr\n(General)')
  xfix : Gain  Gain=xfix  SaturateOnIntegerOverflow=on  OutDataTypeStr=Inherit: Same as input  ParamDataTypeStr=Inherit: Same as input
  x : Outport
  xdot : Outport  Port=2
  ybvel : Outport  Port=3
  wires:
  " *1"/1 -> ODE/1(x)
  xfix/1 -> xdot/1, Discrete-Time Integrator/1
  Discrete-Time Integrator/1 -> *1/1, " *1"/1, x/1
  *1/1 -> uvw/2(x)
  Mtot/1 -> ODE/3(Mtot)
  Ftot/1 -> ODE/2(Ftot)
  yatm/1 -> xdotcorr/3(yatm)
  xdotcorr/1(xdot corrected) -> xfix/1
  Demux/1 -> Sum/1
  uwind/1 -> Demux/1
  uvw/1(ybvel) -> Sum/2, ybvel/1
  Sum/1 -> ODE/5(ybvel*)
  ODE/1(xdot) -> xdotcorr/1(xdot uncorrected)
  yhlp/1 -> xdotcorr/2(yhlp), ODE/4(yhlp), uvw/1(yhlp)
  Demux/2 -> Terminator_1/1

== system RASCAL72_cl/RASCAL-72/fms ==
  FMaero : Inport
  FMprop : Inport  Port=2
  Fgrav : Inport  Port=3
  Fwind : Inport  Port=4
  0 : Subsystem
      mask Display: disp('FMSORT\nM.O. Rauw, October 1997')
  Demux : Demux  Outputs=[3 3]
  Demux1 : Demux  Outputs=[3 3]
  Sum1 : Sum  SaturateOnIntegerOverflow=on  InputSameDT=on  OutDataTypeStr=Inherit: Same as first input
  Sum3 : Sum  Inputs=++++  SaturateOnIntegerOverflow=on  InputSameDT=on  OutDataTypeStr=Inherit: Same as first input
  Ftot : Outport
  Mtot : Outport  Port=2
  wires:
  Fwind/1 -> Sum3/4
  Demux/1 -> Sum3/1
  Sum1/1 -> Mtot/1
  Sum3/1 -> Ftot/1
  Demux1/1 -> Sum3/2
  Fgrav/1 -> Sum3/3
  Demux/2 -> Sum1/1
  Demux1/2 -> Sum1/2
  FMprop/1 -> Demux1/1
  FMaero/1 -> Demux/1

== system RASCAL72_cl/RASCAL-72/fw ==
  x : Inport
  uwind : Inport  Port=2
  -Xw/m : Fcn  Expr=u[16] + u[5]*u[15] - u[6]*u[14]
  -Yw/m : Fcn  Expr=u[17] - u[4]*u[15] + u[6]*u[13]
  -Zw/m : Fcn  Expr=u[18] + u[4]*u[14] - u[5]*u[13]
  0 : Subsystem
      mask Display: disp('FWIND\nM.O. Rauw, Dec. 1996')
  Mux : Mux  Inputs=3
  Mux1 : Mux  Inputs=[12 6]
  gain : Gain  Gain=-m  SaturateOnIntegerOverflow=on  OutDataTypeStr=Inherit: Same as input  ParamDataTypeStr=Inherit: Same as input
  Fwind : Outport
  wires:
  -Zw/m/1 -> Mux/3
  -Xw/m/1 -> Mux/1
  -Yw/m/1 -> Mux/2
  Mux1/1 -> -Xw/m/1, -Zw/m/1, -Yw/m/1
  Mux/1 -> gain/1
  gain/1 -> Fwind/1
  x/1 -> Mux1/1
  uwind/1 -> Mux1/2

== system RASCAL72_cl/RASCAL-72/gr ==
  x : Inport
  yatm : Inport  Port=2
  0 : Subsystem
      mask Display: disp('GRAVITY\nM.O. Rauw, October 1997')
  Mux : Mux  Inputs=3
  Mux1 : Mux  Inputs=[12 5]
  Xgr : Fcn  Expr=-m*u[17]*sin(u[8])
  Ygr : Fcn  Expr=m*u[17]*cos(u[8])*sin(u[9])
  Zgr : Fcn  Expr=m*u[17]*cos(u[8])*cos(u[9])
  Fgrav : Outport
  wires:
  yatm/1 -> Mux1/2
  x/1 -> Mux1/1
  Zgr/1 -> Mux/3
  Mux1/1 -> Zgr/1, Xgr/1, Ygr/1
  Mux/1 -> Fgrav/1
  Ygr/1 -> Mux/2
  Xgr/1 -> Mux/1

== system RASCAL72_cl/RASCAL-72/hlp ==
  x : Inport
  0 : Subsystem
      mask Display: disp('HELP FUNCTIONS\n(often used sines and cosines)\nM.O. Rauw, October 1997')
  Mux : Mux  Inputs=11
  cos alpha : Fcn  Expr=cos(u[2])
  cos beta : Fcn  Expr=cos(u[3])
  cos phi : Fcn  Expr=cos(u[9])
  cos psi : Fcn  Expr=cos(u[7])
  cos theta : Fcn  Expr=cos(u[8])
  sin alpha : Fcn  Expr=sin(u[2])
  sin beta : Fcn  Expr=sin(u[3])
  sin phi : Fcn  Expr=sin(u[9])
  sin psi : Fcn  Expr=sin(u[7])
  sin theta : Fcn  Expr=sin(u[8])
  tan beta : Fcn  Expr=tan(u[3])
  yhlp : Outport
  wires:
  cos phi/1 -> Mux/11
  Mux/1 -> yhlp/1
  sin phi/1 -> Mux/10
  cos theta/1 -> Mux/9
  sin theta/1 -> Mux/8
  cos psi/1 -> Mux/7
  sin psi/1 -> Mux/6
  tan beta/1 -> Mux/5
  sin beta/1 -> Mux/4
  cos beta/1 -> Mux/3
  sin alpha/1 -> Mux/2
  cos alpha/1 -> Mux/1
  x/1 -> cos psi/1, cos phi/1, sin phi/1, cos theta/1, sin theta/1, tan beta/1, cos alpha/1, sin alpha/1, cos beta/1, sin beta/1, sin psi/1

== system RASCAL72_cl/RASCAL-72/out ==
  note: Body-axes accelerations
      | and specific forces
  note: du/dt, dv/dt, dw/dt
      | (output equations!)
  note: Flightpath
      | variables
  x : Inport
  xdot : Inport  Port=2
  yhlp : Inport  Port=3
  Ftot : Inport  Port=4
  Fgrav : Inport  Port=5
  0 : Subsystem
      mask Display: disp('Additional outputs (level 3)\nM.O. Rauw')
  accel : Subsystem  mask(accel){m=GM1(10)}
      mask prompts: m "Mass of the aircraft [kg]:"
      mask help:
      | Body axes accelerations and
      | specific forces.
      mask Display: disp('Accel')
  fp : Subsystem  mask(Flpath){alpha0=x0(2)}
      mask prompts: alpha0 "Initial value of angle of attack, alpha0:"
      mask help: Flightpath related parameters.
      mask Display: disp('flpath')
  uvwdot : Subsystem  mask(uvwdot){}
      mask help: Calculation of du/dt, dv/dt, and dw/dt.
      mask Display: disp('uvwdot')
  yfp : Outport
  yuvw : Outport  Port=2
  yacc : Outport  Port=3
  wires:
  Fgrav/1 -> accel/2(Fgrav)
  x/1 -> uvwdot/1(x), fp/1(x)
  xdot/1 -> uvwdot/2(xdot), fp/2(xdot)
  accel/1(yacc) -> yacc/1
  Ftot/1 -> accel/1(Ftot)
  yhlp/1 -> uvwdot/3(yhlp)
  uvwdot/1(yuvw = [udot; vdot; wdot]) -> yuvw/1
  fp/1(yfp) -> yfp/1

== system RASCAL72_cl/elevator/IIR1 ==
  In : Inport
  Discrete State-Space : DiscreteStateSpace  A=A  B=B  C=C  D=D  InitialCondition=x0  SampleTime=T
  Out : Outport
  wires:
  Discrete State-Space/1 -> Out/1
  In/1 -> Discrete State-Space/1

== system RASCAL72_cl/elevator/IIR2 ==
  In : Inport
  Discrete State-Space : DiscreteStateSpace  A=A  B=B  C=C  D=D  InitialCondition=x0  SampleTime=T
  Out : Outport
  wires:
  Discrete State-Space/1 -> Out/1
  In/1 -> Discrete State-Space/1

== system RASCAL72_cl/elevator/IIR3 ==
  In : Inport
  Discrete State-Space : DiscreteStateSpace  A=A  B=B  C=C  D=D  InitialCondition=x0  SampleTime=T
  Out : Outport
  wires:
  Discrete State-Space/1 -> Out/1
  In/1 -> Discrete State-Space/1

== system RASCAL72_cl/elevator/IIR4 ==
  In : Inport
  Discrete State-Space : DiscreteStateSpace  A=A  B=B  C=C  D=D  InitialCondition=x0  SampleTime=T
  Out : Outport
  wires:
  Discrete State-Space/1 -> Out/1
  In/1 -> Discrete State-Space/1

== system RASCAL72_cl/elevator/t ==

== system RASCAL72_cl/RASCAL-72/ad/0 ==

== system RASCAL72_cl/RASCAL-72/ad/ad1 ==
  x : Inport
  yatm : Inport  Port=2
  0 : Subsystem
      mask Display: disp('AIRDATA1\nM.O. Rauw, October 1997')
  M : Fcn  Expr=u[2]/u[1]
  Mux : Mux  Inputs=[1 12]
  Mux1 : Mux  Inputs=[12 5]
  Mux2 : Mux  Inputs=3
  a : Fcn  Expr=sqrt(401.8743*u[3])
  qdyn : Fcn  Expr=0.5*u[13]*u[1]^2
  yad1 : Outport
  wires:
  yatm/1 -> Mux1/2, a/1
  x/1 -> Mux1/1, Mux/2
  Mux/1 -> M/1
  Mux1/1 -> qdyn/1
  M/1 -> Mux2/2
  a/1 -> Mux2/1, Mux/1
  qdyn/1 -> Mux2/3
  Mux2/1 -> yad1/1

== system RASCAL72_cl/RASCAL-72/ad/ad2 ==
  yatm : Inport
  yad1 : Inport  Port=2
  0 : Subsystem
      mask Display: disp('AIRDATA2\nM.O. Rauw, October 1997')
  Mux : Mux  Inputs=[5 3]
  Mux1 : Mux  Inputs=3
  Vc : Fcn  Expr=sqrt(579000*((1+u[1]/101325)^(1/3.5)-1))
  Ve : Fcn  Expr=sqrt(u[8] * 1.63265)
  qc : Fcn  Expr=u[2] * ((1+0.2*u[7]^2)^3.5-1)
  yad2 : Outport
  wires:
  Mux1/1 -> yad2/1
  qc/1 -> Mux1/1, Vc/1
  Vc/1 -> Mux1/3
  Ve/1 -> Mux1/2
  Mux/1 -> Ve/1, qc/1
  yatm/1 -> Mux/1
  yad1/1 -> Mux/2

== system RASCAL72_cl/RASCAL-72/ad/ad3 ==
  x : Inport
  yatm : Inport  Port=2
  yad1 : Inport  Port=3
  0 : Subsystem
      mask Display: disp('AIRDATA3\nM.O. Rauw, October 1997')
  Mux : Mux  Inputs=3
  Mux1 : Mux  Inputs=[12 5 3]
  Re : Fcn  Expr=(u[13]*u[1])/u[16]
  Tt : Fcn  Expr=u[15] * (1+0.2*u[19]^2)
  cbar : Gain  Gain=cbar  SaturateOnIntegerOverflow=on  OutDataTypeStr=Inherit: Same as input  ParamDataTypeStr=Inherit: Same as input
  yad3 : Outport
  wires:
  cbar/1 -> Mux/3
  Tt/1 -> Mux/1
  Mux/1 -> yad3/1
  Mux1/1 -> Tt/1, Re/1
  Re/1 -> cbar/1, Mux/2
  x/1 -> Mux1/1
  yatm/1 -> Mux1/2
  yad1/1 -> Mux1/3

== system RASCAL72_cl/RASCAL-72/ad/atm ==
  x : Inport
  0 : Subsystem
      mask Display: disp('ATMOSPH\nM.O. Rauw, October 1997')
  Mux : Mux  Inputs=2
  Mux1 : Mux  Inputs=[2 1]
  Mux2 : Mux  Inputs=5
  T : Fcn  Expr=288.15 - 0.0065*u[12]
  g : Fcn  Expr=9.80665*(6371020/(6371020+u[12]))^2
  mu : Fcn  Expr=(1.458*10^(-6)*u[2]^1.5)/(u[2]+110.4)
  ps : Fcn  Expr=101325*(u[2]/288.15)^(u[1]/1.86584)
  rho : Fcn  Expr=u[3]/(287.053*u[2])
  yatm : Outport
  wires:
  mu/1 -> Mux2/4
  Mux2/1 -> yatm/1
  Mux1/1 -> rho/1
  rho/1 -> Mux2/1
  g/1 -> Mux2/5, Mux/1
  T/1 -> Mux2/3, Mux/2
  ps/1 -> Mux2/2, Mux1/2
  Mux/1 -> ps/1, mu/1, Mux1/1
  x/1 -> g/1, T/1

== system RASCAL72_cl/RASCAL-72/ae/0 ==

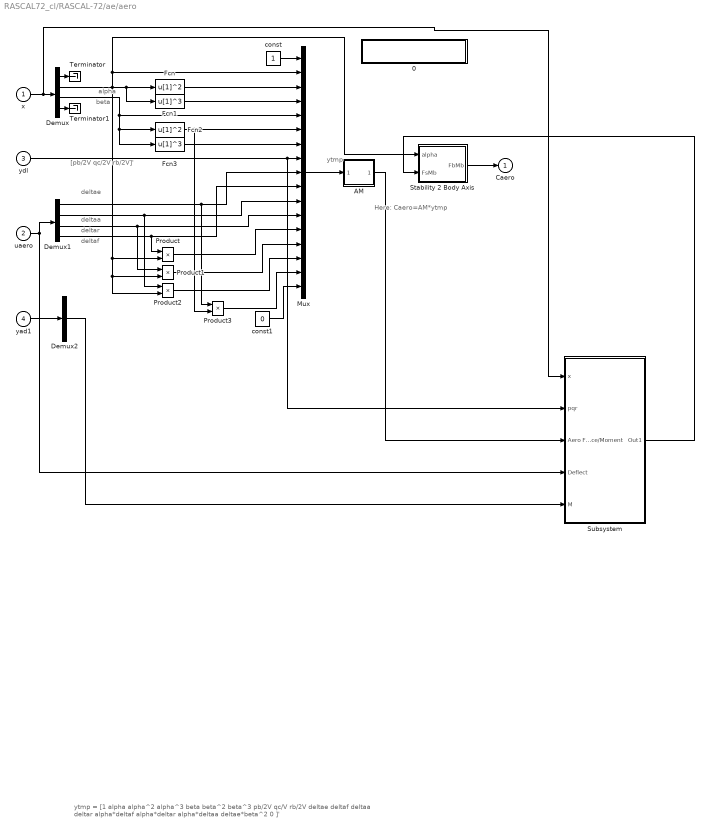
== system RASCAL72_cl/RASCAL-72/ae/aero ==
  note: Here: Caero=AM*ytmp
  note: ytmp
  note: alpha
  note: deltaf
  note: deltar
  note: deltaa
  note: deltae
  note: beta
  note: [pb/2V qc/2V rb/2V]'
  note: ytmp = [1  alpha  alpha^2  alpha^3  beta  beta^2  beta^3  pb/2V  qc/V  rb/2V  deltae
      | deltaf  deltaa  deltar  alpha*deltaf  alpha*deltar  alpha*deltaa  deltae*beta^2  0 ]'
  x : Inport
  uaero : Inport  Port=2
  ydl : Inport  Port=3
  yad1 : Inport  Port=4
  0 : Subsystem
      mask Display: disp('AEROMOD\nM.O. Rauw, October 1997')
  "AM " : Subsystem  mask(State Space){M=AM}
      mask prompts: M "Matrix"
      mask Display: disp('Matrix\nGain')
  Demux : Demux  Outputs=[1 1 1 9]
  Demux1 : Demux
  Demux2 : Demux  Outputs=3
  Fcn : Fcn  Expr=u[1]^2
  Fcn1 : Fcn  Expr=u[1]^3
  Fcn2 : Fcn  Expr=u[1]^2
  Fcn3 : Fcn  Expr=u[1]^3
  Mux : Mux  Inputs=[1 1 1 1 1 1 1 3 1 1 1 1 1 1 1 1 1]
  Product{,1..3} (4 alike) : Product  SaturateOnIntegerOverflow=on  RndMeth=Zero  InputSameDT=on  OutDataTypeStr=Inherit: Same as first input
  Stability 2 Body Axis : Subsystem
  Subsystem : Subsystem
  Terminator : Terminator
  Terminator1 : Terminator
  const : Constant
  const1 : Constant  Value=0
  Caero : Outport
  wires:
  Stability 2 Body Axis/1(FbMb) -> Caero/1
  Mux/1 -> "AM "/1(In1)
  x/1 -> Subsystem/1(x), Demux/1
  Fcn/1 -> Mux/3
  Fcn1/1 -> Mux/4
  uaero/1 -> Demux1/1, Subsystem/4(Deflect)
  Fcn3/1 -> Mux/7
  Product/1 -> Mux/13
  Demux1/3 -> Product1/1, Mux/12
  Demux1/2 -> Product2/1, Mux/11
  Demux/3 -> Fcn3/1, Fcn2/1, Mux/5
  Demux/2 -> Stability 2 Body Axis/1(alpha), Mux/2, Product2/2, Product1/2, Product/2, Fcn1/1, Fcn/1
  Demux1/4 -> Product/1, Mux/10
  Fcn2/1 -> Product3/2, Mux/6
  Product1/1 -> Mux/14
  Product2/1 -> Mux/15
  Product3/1 -> Mux/16
  const/1 -> Mux/1
  const1/1 -> Mux/17
  Demux/1 -> Terminator/1
  Demux/4 -> Terminator1/1
  ydl/1 -> Subsystem/2(pqr), Mux/8
  "AM "/1(Out1) -> Subsystem/3("Aero Force/Moment ")
  Demux1/1 -> Product3/1, Mux/9
  yad1/1 -> Demux2/1
  Demux2/2 -> Subsystem/5(M)
  Subsystem/1(Out1) -> Stability 2 Body Axis/2(FsMb)

== system RASCAL72_cl/RASCAL-72/ae/dl ==
  x : Inport
  0 : Subsystem
      mask Display: disp('DIMLESS\nM.O. Rauw, October 1997')
  Mux : Mux  Inputs=3
  pb/2V : Fcn  Expr=0.5 * u[4] * b / u[1]
  qc/2V : Fcn  Expr=0.5* u[5] * cbar / u[1]
  rb/2V : Fcn  Expr=0.5 * u[6] * b / u[1]
  ydl : Outport
  wires:
  x/1 -> pb/2V/1, rb/2V/1, qc/2V/1
  Mux/1 -> ydl/1
  rb/2V/1 -> Mux/3
  qc/2V/1 -> Mux/2
  pb/2V/1 -> Mux/1

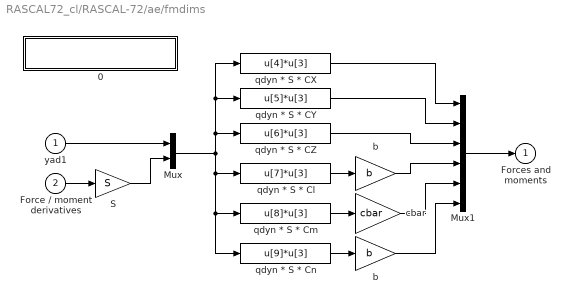
== system RASCAL72_cl/RASCAL-72/ae/fmdims ==
  yad1 : Inport
  Force / moment derivatives : Inport  Port=2
  0 : Subsystem
      mask Display: disp('FMDIMS\nM.O. Rauw, October 1997')
  Mux : Mux  Inputs=[3 6]
  Mux1 : Mux  Inputs=6
  S : Gain  Gain=S  SaturateOnIntegerOverflow=on  OutDataTypeStr=Inherit: Same as input  ParamDataTypeStr=Inherit: Same as input
  b : Gain  Gain=b  SaturateOnIntegerOverflow=on  OutDataTypeStr=Inherit: Same as input  ParamDataTypeStr=Inherit: Same as input
  "b " : Gain  Gain=b  SaturateOnIntegerOverflow=on  OutDataTypeStr=Inherit: Same as input  ParamDataTypeStr=Inherit: Same as input
  cbar : Gain  Gain=cbar  SaturateOnIntegerOverflow=on  OutDataTypeStr=Inherit: Same as input  ParamDataTypeStr=Inherit: Same as input
  qdyn * S * CX : Fcn  Expr=u[4]*u[3]
  qdyn * S * CY : Fcn  Expr=u[5]*u[3]
  qdyn * S * CZ : Fcn  Expr=u[6]*u[3]
  qdyn * S * Cl : Fcn  Expr=u[7]*u[3]
  qdyn * S * Cm : Fcn  Expr=u[8]*u[3]
  qdyn * S * Cn : Fcn  Expr=u[9]*u[3]
  Forces and moments : Outport
  wires:
  b/1 -> Mux1/4
  qdyn * S * CZ/1 -> Mux1/3
  S/1 -> Mux/2
  qdyn * S * CY/1 -> Mux1/2
  qdyn * S * CX/1 -> Mux1/1
  yad1/1 -> Mux/1
  qdyn * S * Cn/1 -> "b "/1
  qdyn * S * Cm/1 -> cbar/1
  qdyn * S * Cl/1 -> b/1
  Mux/1 -> qdyn * S * Cn/1, qdyn * S * Cm/1, qdyn * S * Cl/1, qdyn * S * CY/1, qdyn * S * CX/1, qdyn * S * CZ/1
  Force / moment derivatives/1 -> S/1
  cbar/1 -> Mux1/5
  "b "/1 -> Mux1/6
  Mux1/1 -> Forces and moments/1

== system RASCAL72_cl/RASCAL-72/eqm/0 ==

== system RASCAL72_cl/RASCAL-72/eqm/? ==

== system RASCAL72_cl/RASCAL-72/eqm/ODE ==
  x : Inport
  Ftot : Inport  Port=2
  Mtot : Inport  Port=3
  yhlp : Inport  Port=4
  ybvel* : Inport  Port=5
  0 : Subsystem
      mask Display: disp('12 Ordinary Differential\nEquations (level 4)\nM.O. Rauw')
  Eulerdot : Subsystem  mask(Eulerdot){}
      mask help:
      | Calculation of d(psi)/dt, d(theta)/dt,
      | and d(phi/dt)
      mask Display: disp('psi dot\ntheta dot\nphi dot')
  Mux : Mux  Inputs=[12 3 3 11]
  Mux1 : Mux  Inputs=[3 3 3 3]
  Vabdot : Subsystem  mask(Vabdot){m=GM1(10)}
      mask prompts: m "Mass of the aircraft [kg]:"
      mask help: Calculation of dV/dt, dalpha/dt, dbeta/dt.
      mask Display: disp('V dot\nalpha dot\nbeta dot')
  pqrdot : Subsystem  mask(pqrdot){}
      mask help: Calculation of dp/dt, dq/dt, and dr/dt
      mask Display: disp('p dot\nq dot\nr dot')
  xyHdot : Subsystem  mask(xyHdot){}
      mask help: Calculation of d(xe)/dt, d(ye)/dt, and dH/dt
      mask Display: disp('xe dot\nye dot\nH dot')
  xdot : Outport
  wires:
  Mux1/1 -> xdot/1
  Vabdot/1(yVab) -> Mux1/1
  pqrdot/1(ypqr) -> Mux1/2
  Eulerdot/1(yeul) -> Mux1/3
  xyHdot/1(yxyH) -> Mux1/4
  yhlp/1 -> Mux/4
  ybvel*/1 -> xyHdot/1(ybvel*)
  Mux/1 -> xyHdot/2(uxYH), Eulerdot/1(ueul), Vabdot/1(uVab), pqrdot/1(upqr)
  Ftot/1 -> Mux/2
  Mtot/1 -> Mux/3
  x/1 -> Mux/1

== system RASCAL72_cl/RASCAL-72/eqm/uvw ==
  yhlp : Inport
  x : Inport  Port=2
  0 : Subsystem
      mask Display: disp('UVW\nM.O. Rauw, October 1997')
  Mux : Mux  Inputs=3
  Mux1 : Mux  Inputs=[12 11]
  u : Fcn  Expr=u[1]*u[13]*u[15]
  v : Fcn  Expr=u[1]*u[16]
  w : Fcn  Expr=u[1]*u[14]*u[15]
  ybvel : Outport
  wires:
  Mux/1 -> ybvel/1
  w/1 -> Mux/3
  v/1 -> Mux/2
  u/1 -> Mux/1
  x/1 -> Mux1/1
  yhlp/1 -> Mux1/2
  Mux1/1 -> v/1, w/1, u/1

== system RASCAL72_cl/RASCAL-72/eqm/xdotcorr ==
  xdot uncorrected : Inport
  yhlp : Inport  Port=2
  yatm : Inport  Port=3
  0 : Subsystem
      mask Display: disp('XDOTCORR (General)\nM.O. Rauw, October 1997')
  Demux : Demux  Outputs=12
  Mux1 : Mux  Inputs=12
  Mux2 : Mux  Inputs=[11 1 5]
  beta dot correction : Fcn  Expr=u[12] / (1 - (u[3]*u[13]*b*S*CYbdot)/(4*m))
  xdot corrected : Outport
  wires:
  yhlp/1 -> Mux2/1
  Mux2/1 -> beta dot correction/1
  Mux1/1 -> xdot corrected/1
  xdot uncorrected/1 -> Demux/1
  Demux/3 -> Mux2/2
  Demux/12 -> Mux1/12
  Demux/11 -> Mux1/11
  Demux/10 -> Mux1/10
  Demux/9 -> Mux1/9
  Demux/8 -> Mux1/8
  Demux/7 -> Mux1/7
  Demux/6 -> Mux1/6
  Demux/5 -> Mux1/5
  Demux/4 -> Mux1/4
  Demux/2 -> Mux1/2
  Demux/1 -> Mux1/1
  yatm/1 -> Mux2/3
  beta dot correction/1 -> Mux1/3

== system RASCAL72_cl/RASCAL-72/fms/0 ==

== system RASCAL72_cl/RASCAL-72/fw/0 ==

== system RASCAL72_cl/RASCAL-72/gr/0 ==

== system RASCAL72_cl/RASCAL-72/hlp/0 ==

== system RASCAL72_cl/RASCAL-72/out/0 ==

== system RASCAL72_cl/RASCAL-72/out/accel ==
  Ftot : Inport
  Fgrav : Inport  Port=2
  0 : Subsystem
      mask Display: disp('ACCEL\nM.O. Rauw, October 1997')
  Ax : Fcn  Expr=(u[1]-u[4])/(m*9.80665)
  Ay : Fcn  Expr=(u[2]-u[5])/(m*9.80665)
  Az : Fcn  Expr=(u[3]-u[6])/(m*9.80665)
  Mux : Mux  Inputs=6
  Mux1 : Mux  Inputs=[3 3]
  axk : Fcn  Expr=u[1]/(m*9.80665)
  ayk : Fcn  Expr=u[2]/(m*9.80665)
  azk : Fcn  Expr=u[3]/(m*9.80665)
  yacc : Outport
  wires:
  ayk/1 -> Mux/5
  axk/1 -> Mux/4
  Mux1/1 -> ayk/1, azk/1, axk/1, Ay/1, Ax/1, Az/1
  Ax/1 -> Mux/1
  Ay/1 -> Mux/2
  Az/1 -> Mux/3
  azk/1 -> Mux/6
  Mux/1 -> yacc/1
  Fgrav/1 -> Mux1/2
  Ftot/1 -> Mux1/1

== system RASCAL72_cl/RASCAL-72/out/fp ==
  x : Inport
  xdot : Inport  Port=2
  0 : Subsystem
      mask Display: disp('FLPATH\nM.O. Rauw, October 1997')
  Mux : Mux  Inputs=[12 12]
  Mux1 : Mux
  Phi : Fcn  Expr=u[9]*cos(u[8]-alpha0)
  chi : Fcn  Expr=u[3]+u[7]
  fpa : Fcn  Expr=u[13]/9.80665
  gamma : Fcn  Expr=asin(u[24]/u[1])
  yfp : Outport
  wires:
  xdot/1 -> Mux/2
  x/1 -> Mux/1
  Mux1/1 -> yfp/1
  Phi/1 -> Mux1/4
  chi/1 -> Mux1/3
  fpa/1 -> Mux1/2
  Mux/1 -> gamma/1, fpa/1, Phi/1, chi/1
  gamma/1 -> Mux1/1

== system RASCAL72_cl/RASCAL-72/out/uvwdot ==
  note: V
  note: sin(beta)
  note: cos(beta)
  note: sin(alpha)
  note: cos(alpha)
  note: `
  x : Inport
  xdot : Inport  Port=2
  yhlp : Inport  Port=3
  0 : Subsystem
      mask Display: disp('UVWDOT\nM.O. Rauw, October 1997')
  DeMux : Demux  Outputs=[1 1 1 1 7]
  Demux : Demux  Outputs=[1 11]
  Mux : Mux  Inputs=[1 1 1 1 1 12]
  Mux1 : Mux  Inputs=3
  Terminator : Terminator
  Terminator1 : Terminator
  u dot : Fcn  Expr=u[6]*u[1]*u[3] - u[5]*(u[7]*u[2]*u[3] + u[8]*u[1]*u[4])
  v dot : Fcn  Expr=u[6]*u[4] + u[5]*u[3]*u[8]
  wdot : Fcn  Expr=u[6]*u[2]*u[3] + u[5]*(u[7]*u[1]*u[3] - u[8]*u[2]*u[4])
  yuvw = [udot; vdot; wdot] : Outport
  wires:
  Demux/1 -> Mux/5
  DeMux/4 -> Mux/4
  DeMux/3 -> Mux/3
  yhlp/1 -> DeMux/1
  Mux1/1 -> yuvw = [udot; vdot; wdot]/1
  x/1 -> Demux/1
  DeMux/2 -> Mux/2
  DeMux/1 -> Mux/1
  Mux/1 -> u dot/1, wdot/1, v dot/1
  xdot/1 -> Mux/6
  u dot/1 -> Mux1/1
  v dot/1 -> Mux1/2
  wdot/1 -> Mux1/3
  DeMux/5 -> Terminator/1
  Demux/2 -> Terminator1/1

== system RASCAL72_cl/RASCAL-72/ad/ad1/0 ==

== system RASCAL72_cl/RASCAL-72/ad/ad2/0 ==

== system RASCAL72_cl/RASCAL-72/ad/ad3/0 ==

== system RASCAL72_cl/RASCAL-72/ad/atm/0 ==

== system RASCAL72_cl/RASCAL-72/ae/aero/0 ==

== system RASCAL72_cl/RASCAL-72/ae/aero/AM  ==
  In1 : Inport
  Matrix Gain : StateSpace  A=[]  B=[]  C=[]  D=M  InitialCondition=0
  Out1 : Outport
  wires:
  Matrix Gain/1 -> Out1/1
  In1/1 -> Matrix Gain/1

== system RASCAL72_cl/RASCAL-72/ae/aero/Stability 2 Body Axis ==
  alpha : Inport
  FsMb : Inport  Port=2
  Demux2 : Demux  Outputs=6
  Mux1 : Mux  Inputs=6
  Product{2..5} (4 alike) : Product  SaturateOnIntegerOverflow=on  RndMeth=Zero  InputSameDT=on  OutDataTypeStr=Inherit: Same as first input
  Sum3 : Sum  Inputs=-+  SaturateOnIntegerOverflow=on  InputSameDT=on  OutDataTypeStr=Inherit: Same as first input
  Sum4 : Sum  Inputs=--  SaturateOnIntegerOverflow=on  InputSameDT=on  OutDataTypeStr=Inherit: Same as first input
  cos alpha : Fcn  Expr=cos(u[1])
  sin alpha : Fcn
  FbMb : Outport
  wires:
  FsMb/1 -> Demux2/1
  Mux1/1 -> FbMb/1
  alpha/1 -> cos alpha/1, sin alpha/1
  Sum4/1 -> Mux1/3
  Product5/1 -> Sum4/2
  Product4/1 -> Sum4/1
  Demux2/3 -> Product5/2, Product3/2
  sin alpha/1 -> Product4/1, Product3/1
  Sum3/1 -> Mux1/1
  Product3/1 -> Sum3/2
  Product2/1 -> Sum3/1
  Demux2/1 -> Product4/2, Product2/2
  cos alpha/1 -> Product5/1, Product2/1
  Demux2/4 -> Mux1/4
  Demux2/2 -> Mux1/2
  Demux2/5 -> Mux1/5
  Demux2/6 -> Mux1/6
